simulink model "Direct_MRAC_Ex1"  (R2023a)
settings: Solver=VariableStepAuto  StartTime=0.0  StopTime=5.0  RelTol=1e-3
undefined symbols (not defined in the file): a, am, b, gamma
settings Model: Creator=geokr  LastModifiedBy=geokr

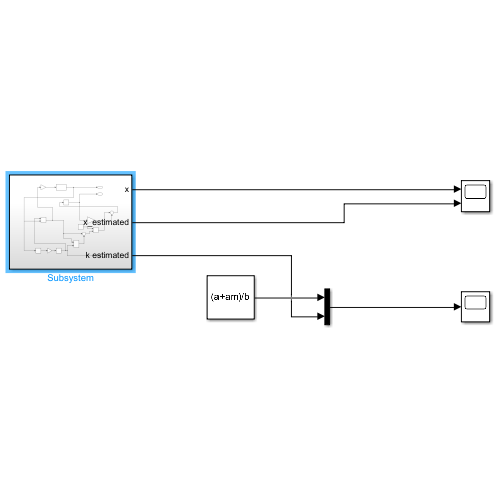
[thumbnail: Simulink's stored preview of the top-level diagram]
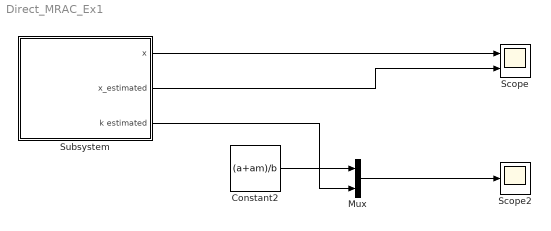
== system Direct_MRAC_Ex1 ==
  Constant2 : Constant  Value=(a+am)/b
  Mux : Mux  Inputs=2
  Scope : Scope  NumInputPorts=2
  Scope2 : Scope
  Subsystem : Subsystem
  wires:
  Mux/1 -> Scope2/1
  Constant2/1 -> Mux/1
  Subsystem/1(x) -> Scope/1
  Subsystem/2(x_estimated) -> Scope/2
  Subsystem/3(k estimated) -> Mux/2

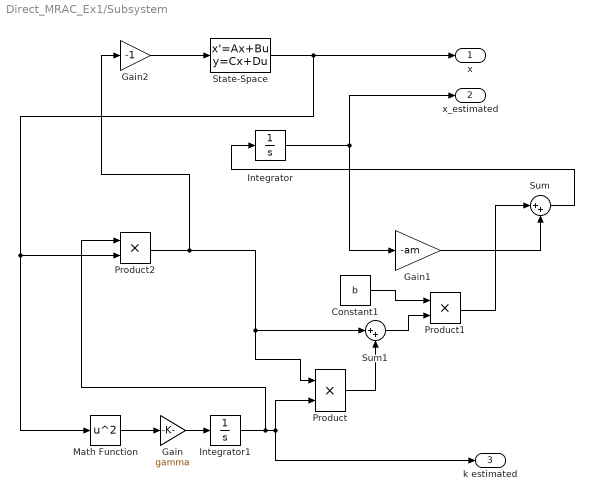
== system Direct_MRAC_Ex1/Subsystem ==
  Constant1 : Constant  Value=b
  Gain : Gain  Gain=gamma
  Gain1 : Gain  Gain=-am
  Gain2 : Gain  Gain=-1
  Integrator : Integrator
  Integrator1 : Integrator
  Math Function : Math  Operator=square
  Product : Product
  Product1 : Product
  Product2 : Product
  State-Space : StateSpace  A=a  B=b  D=0  InitialCondition=20
  Sum : Sum  Inputs=|++
  Sum1 : Sum  Inputs=|++
  x : Outport
  x_estimated : Outport  Port=2
  k estimated : Outport  Port=3
  wires:
  Math Function/1 -> Gain/1
  Gain/1 -> Integrator1/1
  Integrator1/1 -> Product2/1, k estimated/1, Product/2
  Product2/1 -> Gain2/1, Product/1, Sum1/1
  State-Space/1 -> x/1, Product2/2, Math Function/1
  Constant1/1 -> Product1/1
  Product/1 -> Sum1/2
  Sum1/1 -> Product1/2
  Integrator/1 -> x_estimated/1, Gain1/1
  Gain1/1 -> Sum/2
  Gain2/1 -> State-Space/1
  Sum/1 -> Integrator/1
  Product1/1 -> Sum/1
